simulink model "OilT_DD"  (R2016b)
settings: configuration reference "CodeGenConfigSet" (kept outside this file)
values from neighbouring files (symbols this model uses):
  Oil_tiMaxTDefDeb_C = Calibration.Parameter    [init_OilT_DD.m]
  Oil_tiMaxTOKDeb_C = Calibration.Parameter    [init_OilT_DD.m]
  Oil_tiMinTDefDeb_C = Calibration.Parameter    [init_OilT_DD.m]
  Oil_tiMinTOKDeb_C = Calibration.Parameter    [init_OilT_DD.m]
  Oil_tTransfT_CUR = Calibration.Parameter    [init_OilT_DD.m]
  Oil_tTransfT_CURX = Calibration.Parameter    [init_OilT_DD.m]
  Oil_uSRCTMax_C = Calibration.Parameter    [init_OilT_DD.m]
  Oil_uSRCTMin_C = Calibration.Parameter    [init_OilT_DD.m]
undefined symbols (not defined in the file or in its folder): OilT_DD_DT
libraries: CXLib x6
settings Model: Creator=Wollf  LastModifiedBy=wangrui
settings ConfigSetRef: SourceLocation=Base Workspace

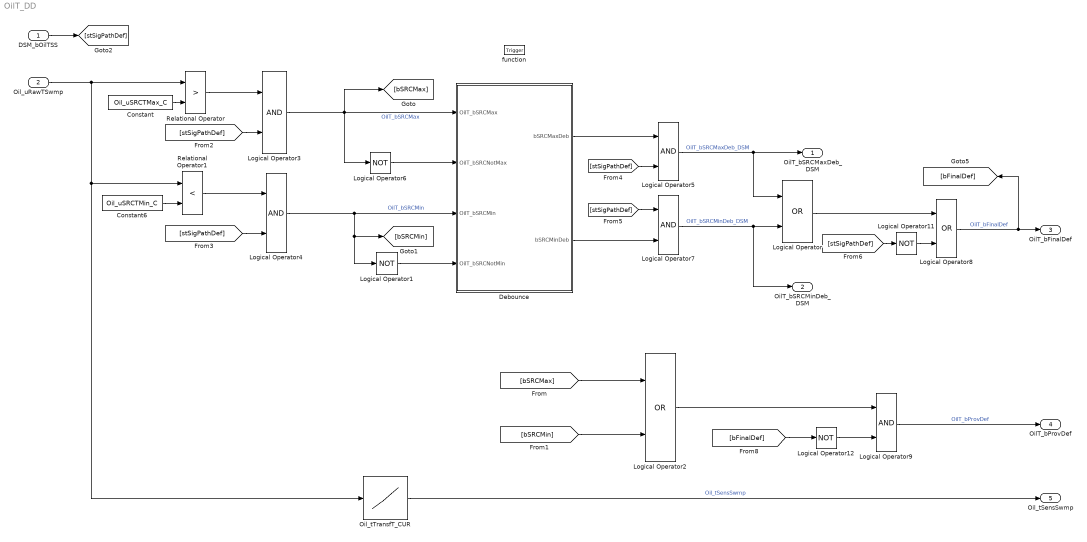
== system OilT_DD ==
  DSM_bOilTSS : Inport  Description=state of FId_OilTSS  OutMin=0  OutMax=1  OutDataTypeStr=boolean
  Oil_uRawTSwmp : Inport  Tag=mv  Description=Raw ADC value of oil temperature sensor  Port=2  OutMin=0  OutMax=5000  OutDataTypeStr=Ad_mv
  function : TriggerPort  TriggerType=function-call  VariantControl=Variant
  Constant : Constant  Value=Oil_uSRCTMax_C
  Constant6 : Constant  Value=Oil_uSRCTMin_C
  Debounce : Subsystem
  Logical Operator : Logic  Operator=OR  AllPortsSameDT=off  OutDataTypeStr=boolean
  Logical Operator{1,6,11..12} (4 alike) : Logic  Operator=NOT  AllPortsSameDT=off  OutDataTypeStr=boolean
  Logical Operator2 : Logic  Operator=OR  AllPortsSameDT=off  OutDataTypeStr=boolean
  Logical Operator{3..5,7,9} (5 alike) : Logic  AllPortsSameDT=off  OutDataTypeStr=boolean
  Logical Operator8 : Logic  Operator=OR  AllPortsSameDT=off  OutDataTypeStr=boolean
  Oil_tTransfT_CUR : Lookup_n-D  NumberOfTableDimensions=1  BreakpointsForDimension1=Oil_tTransfT_CURX  BreakpointsForDimension3=[5, 7]  IndexSearchMethod=Linear search  BeginIndexSearchUsingPreviousIndexResult=on  Table=Oil_tTransfT_CUR  ExtrapMethod=Clip  UseLastTableValue=on  InternalRulePriority=Speed  OutDataTypeStr=Inherit: Inherit via back propagation  RndMeth=Simplest  SaturateOnIntegerOverflow=on
  Relational Operator : RelationalOperator  Operator=>  OutDataTypeStr=boolean  RndMeth=Nearest  InputSameDT=on
  Relational Operator1 : RelationalOperator  Operator=<  OutDataTypeStr=boolean  RndMeth=Nearest  InputSameDT=on
  OilT_bSRCMaxDeb_DSM : Outport  Description=status of OilT_bSRCMaxDeb  OutMin=0  OutMax=1  OutDataTypeStr=boolean
  OilT_bSRCMinDeb_DSM : Outport  Description=status of OilT_bSRCMinDeb  Port=2  OutMin=0  OutMax=1  OutDataTypeStr=boolean
  OilT_bFinalDef : Outport  Description=Status Sensor of the oil temperature finally defect  Port=3  OutMin=0  OutMax=1  OutDataTypeStr=boolean
  OilT_bProvDef : Outport  Description=Status sensor of the oil temperature temporary defect  Port=4  OutMin=0  OutMax=1  OutDataTypeStr=boolean
  Oil_tSensSwmp : Outport  Tag=deg  Description=Sensed value of oil temperature  Port=5  OutMin=-50  OutMax=200  OutDataTypeStr=Temp_deg
  wires:
  Oil_uRawTSwmp/1 -> Oil_tTransfT_CUR/1, Relational Operator1/1, Relational Operator/1
  Oil_tTransfT_CUR/1 -> Oil_tSensSwmp/1  "Oil_tSensSwmp"
  Constant/1 -> Relational Operator/2
  Logical Operator3/1 -> Debounce/1(OilT_bSRCMax), [bSRCMax], Logical Operator6/1  "OilT_bSRCMax"
  Constant6/1 -> Relational Operator1/2
  Logical Operator4/1 -> Logical Operator1/1, [bSRCMin], Debounce/3(OilT_bSRCMin)  "OilT_bSRCMin"
  Logical Operator5/1 -> OilT_bSRCMaxDeb_DSM/1, Logical Operator/1  "OilT_bSRCMaxDeb_DSM"
  Logical Operator7/1 -> OilT_bSRCMinDeb_DSM/1, Logical Operator/2  "OilT_bSRCMinDeb_DSM"
  [bSRCMax] -> Logical Operator2/1
  [bSRCMin] -> Logical Operator2/2
  Relational Operator/1 -> Logical Operator3/1
  [stSigPathDef] -> Logical Operator3/2
  Relational Operator1/1 -> Logical Operator4/1
  [stSigPathDef] -> Logical Operator4/2
  [stSigPathDef] -> Logical Operator5/2
  [stSigPathDef] -> Logical Operator7/1
  Logical Operator/1 -> Logical Operator8/1
  [stSigPathDef] -> Logical Operator11/1
  Logical Operator2/1 -> Logical Operator9/1
  [bFinalDef] -> Logical Operator12/1
  Logical Operator8/1 -> OilT_bFinalDef/1, [bFinalDef]  "OilT_bFinalDef"
  Logical Operator9/1 -> OilT_bProvDef/1  "OilT_bProvDef"
  Logical Operator11/1 -> Logical Operator8/2
  Logical Operator12/1 -> Logical Operator9/2
  Logical Operator6/1 -> Debounce/2(OilT_bSRCNotMax)
  Logical Operator1/1 -> Debounce/4(OilT_bSRCNotMin)
  Debounce/1(bSRCMaxDeb) -> Logical Operator5/1
  Debounce/2(bSRCMinDeb) -> Logical Operator7/2
  DSM_bOilTSS/1 -> [stSigPathDef]

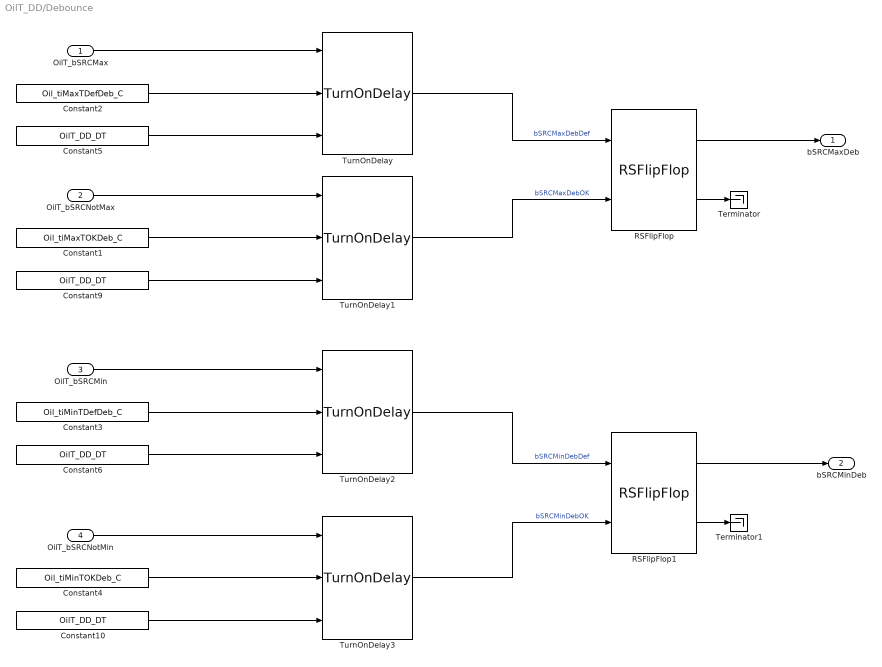
== system OilT_DD/Debounce ==
  OilT_bSRCMax : Inport
  OilT_bSRCNotMax : Inport  Port=2
  OilT_bSRCMin : Inport  Port=3
  OilT_bSRCNotMin : Inport  Port=4
  Constant1 : Constant  Value=Oil_tiMaxTOKDeb_C
  Constant{5..6,9..10} (4 alike) : Constant  Value=OilT_DD_DT  OutDataTypeStr=Inherit: Inherit via back propagation
  Constant2 : Constant  Value=Oil_tiMaxTDefDeb_C
  Constant3 : Constant  Value=Oil_tiMinTDefDeb_C
  Constant4 : Constant  Value=Oil_tiMinTOKDeb_C
  RSFlipFlop : CXLib/RSFlipFlop
  RSFlipFlop1 : CXLib/RSFlipFlop
  Terminator : Terminator
  Terminator1 : Terminator
  TurnOnDelay{,1..3} (4 alike) : CXLib/TurnOnDelay
  bSRCMaxDeb : Outport
  bSRCMinDeb : Outport  Port=2
  wires:
  Constant10/1 -> TurnOnDelay3/3
  Constant6/1 -> TurnOnDelay2/3
  Constant9/1 -> TurnOnDelay1/3
  Constant5/1 -> TurnOnDelay/3
  RSFlipFlop1/1 -> bSRCMinDeb/1
  RSFlipFlop/1 -> bSRCMaxDeb/1
  TurnOnDelay1/1 -> RSFlipFlop/2  "bSRCMaxDebOK"
  Constant3/1 -> TurnOnDelay2/2
  Constant1/1 -> TurnOnDelay1/2
  Constant2/1 -> TurnOnDelay/2
  TurnOnDelay/1 -> RSFlipFlop/1  "bSRCMaxDebDef"
  OilT_bSRCNotMax/1 -> TurnOnDelay1/1
  OilT_bSRCMin/1 -> TurnOnDelay2/1
  TurnOnDelay2/1 -> RSFlipFlop1/1  "bSRCMinDebDef"
  OilT_bSRCNotMin/1 -> TurnOnDelay3/1
  TurnOnDelay3/1 -> RSFlipFlop1/2  "bSRCMinDebOK"
  Constant4/1 -> TurnOnDelay3/2
  RSFlipFlop/2 -> Terminator/1
  RSFlipFlop1/2 -> Terminator1/1
  OilT_bSRCMax/1 -> TurnOnDelay/1
